simulink model "Pengmod"  (R2018b)
settings: Solver=ode45  StartTime=0.0  StopTime=1  RelTol=1e-3  EnableMultiTasking=on
libraries: powerlib x15, powerlib_meascontrol x2
settings Model: Creator=Kumar Pranshu  LastModifiedBy=Hp
settings DataIOCC: LimitDataPoints=on  SaveFormat=Array
settings OptimizationCC: LifeSpan=inf
settings DebuggingCC: SolverPrmCheckMsg=warning  SFUnexpectedBacktrackingDiag=warning  SFNoUnconditionalDefaultTransitionDiag=warning  SFExecutionAtInitializationDiag=none
settings HardwareCC: ProdBitPerPointer=32  ProdBitPerSizeT=32  ProdBitPerPtrDiffT=32  ProdLargestAtomicFloat=None  ProdIntDivRoundTo=Undefined  ProdEndianess=Unspecified  ProdWordSize=32  ProdHWDeviceType=32-bit Generic
settings ModelReferenceCC: PropagateSignalLabelsOutOfModel=off
settings SFSimCC: SimUseLocalCustomCode=off
settings RTWCC: RTWUseLocalCustomCode=off
settings CodeAppCC: StateflowObjectComments=on
settings GRTTargetCC: TargetLangStandard=C89/C90 (ANSI)  GeneratePreprocessorConditionals=Disable all
settings ConfigComp: CovMetricSettings=dw  CovHtmlReporting=on  CovSaveCumulativeToWorkspaceVar=on  CovSaveSingleToWorkspaceVar=on  CovExternalEMLEnable=off  CovSFcnEnable=off
settings SimscapeCC: SimscapeNormalizeSystem=off

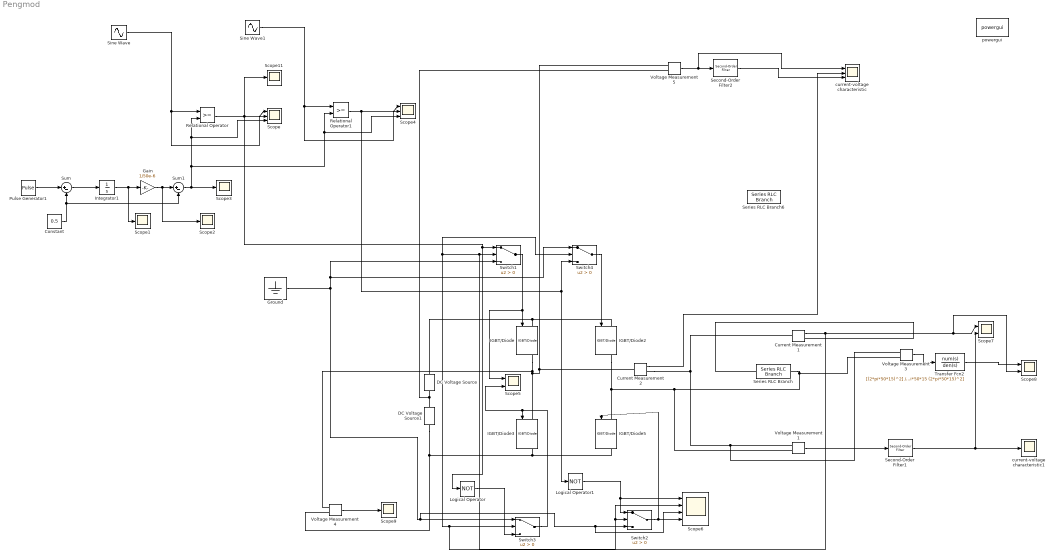
== system Pengmod ==
  Constant : Constant  Value=0.5
  Current Measurement1 : powerlib/Measurements/Current Measurement  PhasorSimulation=off  OutputType=Complex  PSBequivalent=0
      settings: SourceProductName=Simscape Electrical
  Current Measurement2 : powerlib/Measurements/Current Measurement  PhasorSimulation=off  OutputType=Complex  PSBequivalent=0
      settings: SourceProductName=Simscape Electrical
  DC Voltage Source : powerlib/Electrical Sources/DC Voltage Source  Amplitude=165  Measurements=None
      settings: SourceProductName=Simscape Electrical
  DC Voltage Source1 : powerlib/Electrical Sources/DC Voltage Source  Amplitude=165  Measurements=None
      settings: SourceProductName=Simscape Electrical
  Gain : Gain  Gain=1/50e-6
  Ground : Ground
  IGBT/Diode{,2..3,5} (4 alike) : powerlib/Power Electronics/IGBT//Diode  Ron=1e-3  Rs=1e9  Cs=47e-9  Measurements=on
      settings: SourceProductName=Simscape Electrical
  Integrator1 : Integrator
  Logical Operator : Logic  Operator=NOT  Inputs=1  AllPortsSameDT=off  OutDataTypeStr=boolean
  Logical Operator1 : Logic  Operator=NOT  Inputs=1  AllPortsSameDT=off  OutDataTypeStr=boolean
  Pulse Generator1 : DiscretePulseGenerator  PulseType=Time based  Period=200e-6  PulseWidth=50
  Relational Operator : RelationalOperator  OutDataTypeStr=boolean  RndMeth=Nearest
  Relational Operator1 : RelationalOperator  OutDataTypeStr=boolean  RndMeth=Nearest
  Scope : Scope  NumInputPorts=3
  Scope{1..3,9,11} (5 alike) : Scope
  Scope4 : Scope  NumInputPorts=3
  Scope5 : Scope  NumInputPorts=2
  Scope6 : Scope  NumInputPorts=4
  Scope7 : Scope  NumInputPorts=2
  Scope8 : Scope  NumInputPorts=2
  Second-Order Filter1 : powerlib_meascontrol/Filters/Second-Order Filter  FilterType=Lowpass  Fo=1000  Zeta=0.707  Ts=0  Initialize=on  Vac_Init="[0,  0,  1000]"  Vdc_Init=0  PlotResponse=off  FreqRange=[0, 500, 1]
      settings: SourceProductName=Simscape Electrical  SourceProductBaseCode=PS
  Second-Order Filter2 : powerlib_meascontrol/Filters/Second-Order Filter  FilterType=Lowpass  Fo=1000  Zeta=0.707  Ts=0  Initialize=on  Vac_Init="[0,  0,  1000]"  Vdc_Init=0  PlotResponse=off  FreqRange=[0, 500, 1]
      settings: SourceProductName=Simscape Electrical  SourceProductBaseCode=PS
  Series RLC Branch : powerlib/Elements/Series RLC Branch  LConnTagsString=__new0  RConnTagsString=__new0  BranchType=RL  Resistance=25  Inductance=250/(100*3.14)  SetiL0=off  InitialCurrent=0  Capacitance=0  Setx0=off  InitialVoltage=0  Measurements=None
      settings: SourceProductName=Simscape Electrical
  Series RLC Branch6 : powerlib/Elements/Series RLC Branch  LConnTagsString=__new0  RConnTagsString=__new0  BranchType=C  Resistance=10  Inductance=10/(2*pi*50)  SetiL0=off  InitialCurrent=0  Capacitance=100e-6  Setx0=off  InitialVoltage=0  Measurements=None
      settings: SourceProductName=Simscape Electrical
  Sine Wave : Sin  Amplitude=0.4  Frequency=2*pi*50  SampleTime=0
  Sine Wave1 : Sin  Amplitude=0.4  Frequency=2*pi*50  Phase=pi  SampleTime=0
  Sum : Sum  Inputs=|+-
  Sum1 : Sum  Inputs=|+-
  Switch{1..4} (4 alike) : Switch  Criteria=u2 > Threshold
  Transfer Fcn2 : TransferFcn  Numerator=[(2*pi*50*15)^2]  Denominator=[1 (1/0.707)*2*pi*50*15 (2*pi*50*15)^2]
  Voltage Measurement{1,3..5} (4 alike) : powerlib/Measurements/Voltage Measurement  PhasorSimulation=off  OutputType=Complex  PSBequivalent=0
      settings: SourceProductName=Simscape Electrical
  current-voltage characteristic : Scope  NumInputPorts=3
  current-voltage characteristic1 : Scope
  powergui : powerlib/powergui  Priority=1  SimulationMode=Continuous  SampleTime=50e-6  frequency=60  Iterations=50  frequencyindice=0  Pbase=100e6  ErrMax=1e-4  UnitsV=kV  UnitsW=MW  buscounter=0  FunctionMessages=off  echomessages=off  EnableUseOfTLC=off  CurrentSourceSwitches=off  DisableSnubberDevices=off  DisableRonSwitches=off  DisableVfSwitches=off  DisplayEquations=off  SolverType=Tustin  Interpol=off  ExternalGateDelay=off  methode=off  Ts=0  x0status=blocks  SPID=off  SwTol=0  HookPort=off  RestoreLinks=warning  ResistiveCurrentMeasurement=off  Frange=[0:2:500]  Ylog=off  Xlog=on  ShowGrid=off  save=off  variable=ZData  structure=current  ZoomFFT=off  StartTime=0.0  cycles=1  DisplayStyle=1  fundamental=50  FreqAxis=off  MaxFrequency=1000  frequencyindicesteady=1  RmsSteady=1  display=off
  wires:
  Sine Wave/1 -> Scope/2, Relational Operator/1
  Integrator1/1 -> Scope1/1, Gain/1
  Pulse Generator1/1 -> Sum/1
  Sum/1 -> Integrator1/1
  Constant/1 -> Sum1/2, Sum/2
  Gain/1 -> Scope2/1, Sum1/1
  Sine Wave1/1 -> Scope4/2, Relational Operator1/1
  Sum1/1 -> Scope3/1, Scope4/3, Relational Operator1/2, Scope/3, Relational Operator/2
  Voltage Measurement4/1 -> Scope9/1
  Logical Operator/1 -> Switch3/3
  Logical Operator1/1 -> Switch2/1, Scope6/1
  Relational Operator/1 -> Scope11/1, Switch1/1, Logical Operator/1, Scope/1
  Relational Operator1/1 -> Scope4/1, Switch4/3, Logical Operator1/1
  Voltage Measurement5/1 -> Second-Order Filter2/1, current-voltage characteristic/1
  Current Measurement2/1 -> current-voltage characteristic/2
  Voltage Measurement1/1 -> Second-Order Filter1/1
  Second-Order Filter1/1 -> Scope7/2, current-voltage characteristic1/1
  Voltage Measurement3/1 -> Transfer Fcn2/1
  Transfer Fcn2/1 -> Scope8/1
  Second-Order Filter2/1 -> current-voltage characteristic/3
  Switch3/1 -> Scope5/2, IGBT/Diode3/1
  Switch2/1 -> IGBT/Diode5/1, Scope6/4
  Switch4/1 -> IGBT/Diode2/1
  Ground/1 -> Switch1/3, Switch4/1, Scope6/3, Switch2/3, Switch3/1
  Current Measurement1/1 -> Scope6/2, Switch2/2, Switch3/2, Switch4/2, Switch1/2, Scope8/2, Scope7/1
  Switch1/1 -> Scope5/1, IGBT/Diode/1
  connections:
  IGBT/Diode2/LConn1 -- IGBT/Diode/LConn1 -- DC Voltage Source/RConn1
  Voltage Measurement4/LConn2 -- DC Voltage Source1/LConn1 -- IGBT/Diode5/RConn1 -- IGBT/Diode3/RConn1
  Voltage Measurement4/LConn1 -- IGBT/Diode/RConn1 -- IGBT/Diode3/LConn1 -- Voltage Measurement5/LConn1 -- Current Measurement2/LConn1
  Current Measurement2/RConn1 -- Current Measurement1/LConn1 -- Voltage Measurement1/LConn1 -- Voltage Measurement3/LConn1
  Series RLC Branch/LConn1 -- Current Measurement1/RConn1
  DC Voltage Source/LConn1 -- DC Voltage Source1/RConn1 -- Voltage Measurement5/LConn2
  Voltage Measurement3/LConn2 -- IGBT/Diode2/RConn1 -- IGBT/Diode5/LConn1 -- Voltage Measurement1/LConn2 -- Series RLC Branch/RConn1
